simulink model "Final_Model"  (R2019a)
settings: Solver=FixedStepDiscrete  StartTime=0.0  StopTime=0.05  RelTol=1e-3
undefined symbols (not defined in the file): Acid, Lead, SampleTime
libraries: powerlib x26, electricdrivelib x1
settings Model: Creator=ryusl  LastModifiedBy=ryusl

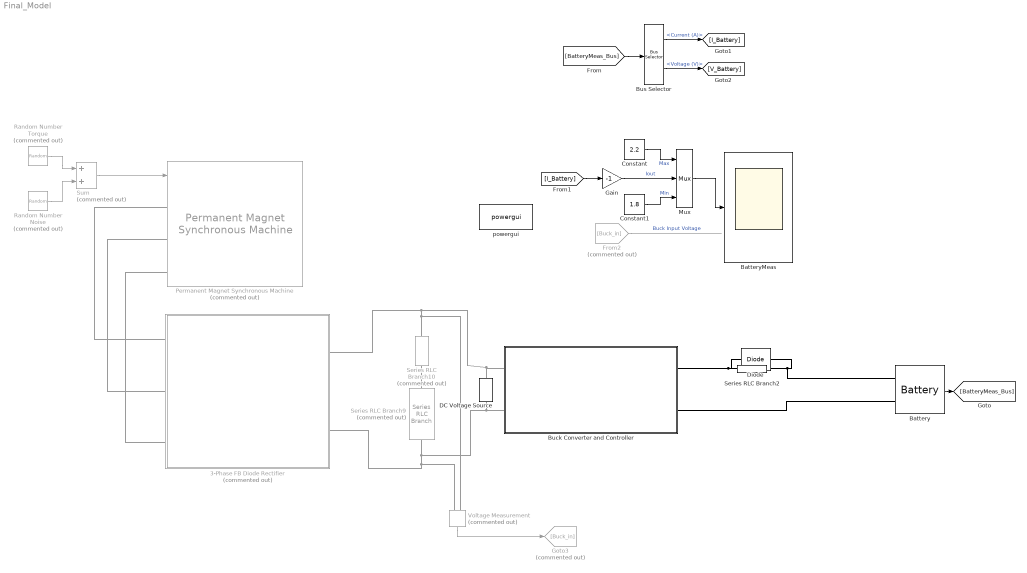
== system Final_Model ==
  3-Phase FB Diode Rectifier : Subsystem  Commented=on
  Battery : electricdrivelib/Extra Sources/Battery  BatType=Lead-Acid  ShowTempParam=off  ThermalPreset=no  ShowAgeParam=off  NomV=24  NomQ=13  SOC=50  Batt_Tr=10  PresetModel=on  MaxQ=13.5417  MinV=18  FullV=26.1316  Dis_rate=2.6  R=0.018462  Normal_OP=4.0336  expZone="[24.4342    0.0433333]"  current=[6.5 13 32.5]  Units=Time  Tci=20  NomT=20  T2=-30  MaxQ2=4.8  FullV2=7.1  Normal_OP2=5.655  expZone2="[6.58           1]"  Rca=0.6  ti=2000  Dp=0  Neq0=0  Tsim=1e6  Ta1=25  Qeol=5.4*0.9  Reol=0.013333*1.2  Char_age=[2.3478, 3]  Dis_age=[2.3478, 10]  N1=1500  N2=10500  N3=1000  N4=1400  Ta2=45  N5=950
  BatteryMeas : Scope
  Buck Converter and Controller : Subsystem
  Bus Selector : BusSelector  OutputSignals=Current (A),Voltage (V)
  Constant : Constant  Value=2.2
  Constant1 : Constant  Value=1.8
  DC Voltage Source : powerlib/Electrical Sources/DC Voltage Source  Amplitude=100  Measurements=None
      settings: SourceProductName=Simscape Electrical
  Diode : powerlib/Power Electronics/Diode  Ron=0.001  Lon=0  Vf=0.3  IC=0  UseSnubber=0  Rs=0  Cs=0  Measurements=off
  From2 : From  Commented=on  GotoTag=Buck_in
  Gain : Gain  Gain=-1
  Goto3 : Goto  Commented=on  GotoTag=Buck_in
  Mux : Mux  Inputs=3
  Permanent Magnet Synchronous Machine : powerlib/Machines/Permanent Magnet Synchronous Machine  Commented=on  NbPhases=3  FluxDistribution=Sinusoidal  RotorType=Round  MechanicalLoad=Torque Tm  PresetModel=No  ShowDetailedParameters=on  MeasurementBus=on  Resistance=10.58  Inductance=8.5e-3  dqInductances=[8.5e-3,8.5e-3]  La=16.7e-3  MachineConstant=Voltage Constant (V_peak L-L / krpm)  Flux=0.60646  VoltageCst=110  TorqueCst=0.90969  Flat=120  Mechanical=[0.00027 0.005024 1 0]  PolePairs=4  InitialConditions=[100,0, 0,0]  InitialConditions5ph=[0 0 0 0 0 0]  TsPowergui=0  TsBlock=-1  RefAngle=90 degrees behind phase A axis (modified Park)
  Random Number Noise : RandomNumber  Commented=on  Variance=0.1  SampleTime=1e-3
  Random Number Torque : RandomNumber  Commented=on  Mean=-1.6  Variance=0.05  SampleTime=0.1
  Series RLC Branch10 : powerlib/Elements/Series RLC Branch  Commented=on  LConnTagsString=__new0  RConnTagsString=__new0  BranchType=R  Resistance=1e-3  Inductance=1e-3  SetiL0=off  InitialCurrent=0  Capacitance=1e-6  Setx0=off  InitialVoltage=0  Measurements=None
  Series RLC Branch2 : powerlib/Elements/Series RLC Branch  LConnTagsString=__new0  RConnTagsString=__new0  BranchType=R  Resistance=1e6  Inductance=1e-3  SetiL0=off  InitialCurrent=0  Capacitance=1e-6  Setx0=off  InitialVoltage=0  Measurements=None
  Series RLC Branch9 : powerlib/Elements/Series RLC Branch  Commented=on  LConnTagsString=__new0  RConnTagsString=__new0  BranchType=C  Resistance=1e6  Inductance=1e-3  SetiL0=off  InitialCurrent=0  Capacitance=56e-6  Setx0=on  InitialVoltage=0  Measurements=None
  Sum : Sum  Commented=on  Inputs=+|+
  Voltage Measurement : powerlib/Measurements/Voltage Measurement  Commented=on  PhasorSimulation=off  OutputType=Complex  PSBequivalent=0
      settings: SourceProductName=Simscape Electrical
  powergui : powerlib/powergui  Priority=1  SimulationMode=Discrete  SampleTime=SampleTime  frequency=60  Iterations=50  frequencyindice=0  Pbase=100e6  ErrMax=1e-4  UnitsV=kV  UnitsW=MW  buscounter=0  FunctionMessages=off  echomessages=off  EnableUseOfTLC=off  CurrentSourceSwitches=off  DisableSnubberDevices=off  DisableRonSwitches=off  DisableVfSwitches=off  DisplayEquations=off  AutomaticDiscreteSolvers=off  SolverType=Tustin/Backward Euler (TBE)  Interpol=off  ExternalGateDelay=off  methode=off  Ts=100  x0status=blocks  SPID=on  SwTol=0  HookPort=off  NonlinearTolerance=1e-4  nMaxIteration=100  ContinueOnMaxIteration=off  RestoreLinks=warning  ResistiveCurrentMeasurement=off  Frange=[0:2:500]  Ylog=off  Xlog=on  ShowGrid=off  save=off  variable=ZData  structure=0  ZoomFFT=off  StartTime=0.0  cycles=1  DisplayStyle=1  fundamental=60  FreqAxis=off  MaxFrequency=1000  frequencyindicesteady=1  RmsSteady=1  display=off
      settings: SourceProductName=Simscape Electrical
  wires:
  Random Number Torque/1 -> Sum/1
  Random Number Noise/1 -> Sum/2
  Sum/1 -> Permanent Magnet Synchronous Machine/1
  Battery/1 -> [BatteryMeas_Bus]
  [BatteryMeas_Bus] -> Bus Selector/1
  Bus Selector/1 -> [I_Battery]  "<Current (A)>"
  Bus Selector/2 -> [V_Battery]  "<Voltage (V)>"
  Constant/1 -> Mux/1  "Max"
  Constant1/1 -> Mux/3  "Min"
  Mux/1 -> BatteryMeas/1
  [I_Battery] -> Gain/1
  Gain/1 -> Mux/2  "Iout"
  Voltage Measurement/1 -> Goto3/1
  From2/1 -> ?  "Buck Input Voltage"
  connections:
  Series RLC Branch10/RConn1 -- Series RLC Branch9/LConn1
  3-Phase FB Diode Rectifier/RConn1 -- DC Voltage Source/RConn1 -- Buck Converter and Controller/LConn1 -- Voltage Measurement/LConn1 -- Series RLC Branch10/LConn1
  3-Phase FB Diode Rectifier/RConn2 -- Voltage Measurement/LConn2 -- DC Voltage Source/LConn1 -- Buck Converter and Controller/LConn2 -- Series RLC Branch9/RConn1
  Buck Converter and Controller/RConn2 -- Battery/LConn2
  Permanent Magnet Synchronous Machine/LConn1 -- 3-Phase FB Diode Rectifier/LConn1
  Permanent Magnet Synchronous Machine/LConn2 -- 3-Phase FB Diode Rectifier/LConn2
  Permanent Magnet Synchronous Machine/LConn3 -- 3-Phase FB Diode Rectifier/LConn3
  Series RLC Branch2/LConn1 -- Diode/RConn1 -- Battery/LConn1
  Series RLC Branch2/RConn1 -- Diode/LConn1 -- Buck Converter and Controller/RConn1

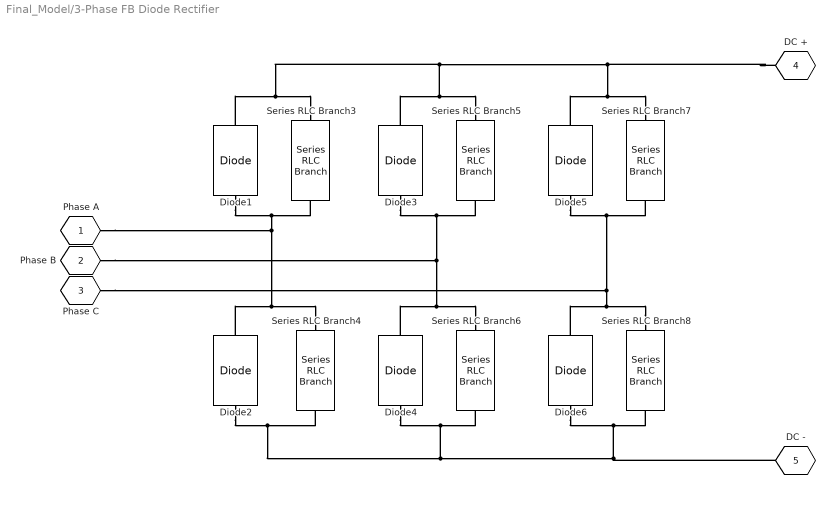
== system Final_Model/3-Phase FB Diode Rectifier ==
  Diode{1..6} (6 alike) : powerlib/Power Electronics/Diode  Ron=Ron  Lon=0  Vf=Vf  IC=0  UseSnubber=0  Rs=0  Cs=0  Measurements=off
  Series RLC Branch{3..8} (6 alike) : powerlib/Elements/Series RLC Branch  LConnTagsString=__new0  RConnTagsString=__new0  BranchType=R  Resistance=1e6  Inductance=1e-3  SetiL0=off  InitialCurrent=0  Capacitance=1e-6  Setx0=off  InitialVoltage=0  Measurements=None
  Phase A : PMIOPort  Tag=PMCPort  Side=Left
  Phase B : PMIOPort  Tag=PMCPort  Port=2  Side=Left
  Phase C : PMIOPort  Tag=PMCPort  Port=3  Side=Left
  DC + : PMIOPort  Tag=PMCPort  Port=4  Side=Right
  DC - : PMIOPort  Tag=PMCPort  Port=5  Side=Right
  connections:
  Diode4/RConn1 -- Phase B/RConn1 -- Diode3/LConn1 -- Series RLC Branch5/RConn1 -- Series RLC Branch6/LConn1
  Diode5/RConn1 -- DC +/RConn1 -- Diode3/RConn1 -- Series RLC Branch5/LConn1 -- Series RLC Branch3/LConn1 -- Diode1/RConn1 -- Series RLC Branch7/LConn1
  Diode2/RConn1 -- Phase A/RConn1 -- Diode1/LConn1 -- Series RLC Branch3/RConn1 -- Series RLC Branch4/LConn1
  Series RLC Branch6/RConn1 -- Diode4/LConn1 -- Diode2/LConn1 -- Series RLC Branch4/RConn1 -- DC -/RConn1 -- Diode6/LConn1 -- Series RLC Branch8/RConn1
  Series RLC Branch8/LConn1 -- Phase C/RConn1 -- Diode5/LConn1 -- Series RLC Branch7/RConn1 -- Diode6/RConn1

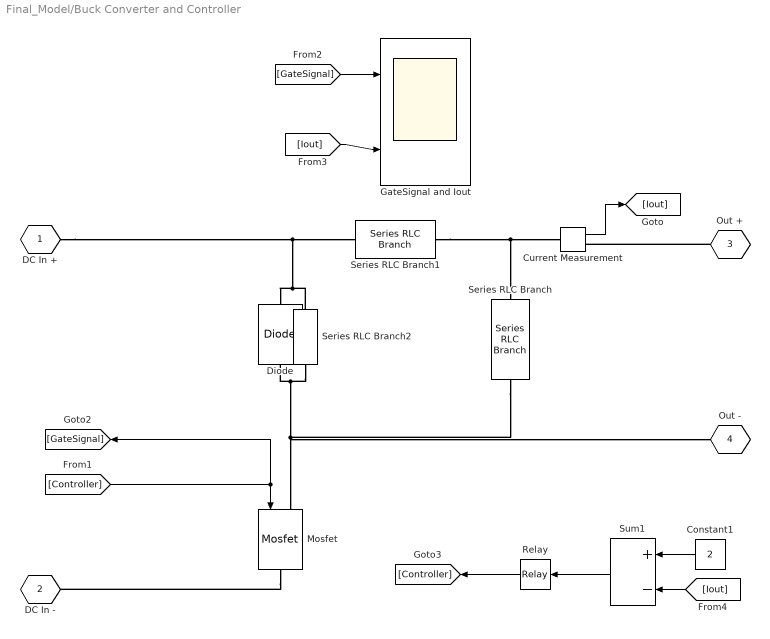
== system Final_Model/Buck Converter and Controller ==
  Constant1 : Constant  Value=2
  Current Measurement : powerlib/Measurements/Current Measurement  PhasorSimulation=off  OutputType=Complex  PSBequivalent=0
      settings: SourceProductName=Simscape Electrical
  Diode : powerlib/Power Electronics/Diode  Ron=0.001  Lon=0  Vf=1  IC=0  UseSnubber=0  Rs=0  Cs=0  Measurements=off
  GateSignal and Iout : Scope  NumInputPorts=2
  Mosfet : powerlib/Power Electronics/Mosfet  Ron=1  Lon=0  Rd=0.01  Vfd=0.3  IC=0  Rs=500  Cs=inf  Measurements=off
  Relay : Relay  OnSwitchValue=0.1  OffSwitchValue=-0.1
  Series RLC Branch : powerlib/Elements/Series RLC Branch  LConnTagsString=__new0  RConnTagsString=__new0  BranchType=RC  Resistance=5e-3  Inductance=1e-9  SetiL0=off  InitialCurrent=0  Capacitance=14.1e-6  Setx0=on  InitialVoltage=0  Measurements=None
  Series RLC Branch1 : powerlib/Elements/Series RLC Branch  LConnTagsString=__new0  RConnTagsString=__new0  BranchType=RL  Resistance=0.379  Inductance=1.5e-3  SetiL0=off  InitialCurrent=0  Capacitance=1e-6  Setx0=off  InitialVoltage=0  Measurements=None
  Series RLC Branch2 : powerlib/Elements/Series RLC Branch  LConnTagsString=__new0  RConnTagsString=__new0  BranchType=R  Resistance=1e6  Inductance=1e-3  SetiL0=off  InitialCurrent=0  Capacitance=1e-6  Setx0=off  InitialVoltage=0  Measurements=None
  Sum1 : Sum  Inputs=+-
  DC In + : PMIOPort  Tag=PMCPort  Side=Left
  DC In - : PMIOPort  Tag=PMCPort  Port=2  Side=Left
  Out + : PMIOPort  Tag=PMCPort  Port=3  Side=Right
  Out - : PMIOPort  Tag=PMCPort  Port=4  Side=Right
  wires:
  [Controller] -> [GateSignal], Mosfet/1
  Current Measurement/1 -> [Iout]
  [GateSignal] -> GateSignal and Iout/1
  [Iout] -> GateSignal and Iout/2
  Relay/1 -> [Controller]
  Constant1/1 -> Sum1/1
  [Iout] -> Sum1/2
  Sum1/1 -> Relay/1
  connections:
  Series RLC Branch2/RConn1 -- Diode/LConn1 -- Series RLC Branch/RConn1 -- Out -/RConn1 -- Mosfet/LConn1
  Series RLC Branch1/RConn1 -- Current Measurement/LConn1 -- Series RLC Branch/LConn1
  DC In +/RConn1 -- Series RLC Branch1/LConn1 -- Diode/RConn1 -- Series RLC Branch2/LConn1
  Mosfet/RConn1 -- DC In -/RConn1
  Out +/RConn1 -- Current Measurement/RConn1
